simulink model "chap7_4sim"  (Simulink 3.00)
settings: Solver=ode45  StartTime=0.0  StopTime=50  FixedStep=0.00001  RelTol=1e-3
settings Model: LastModifiedBy=liu

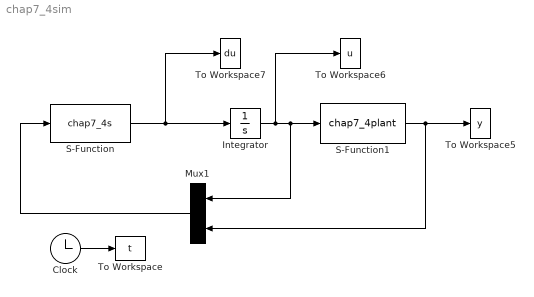
== system chap7_4sim ==
  Clock : Clock
  Integrator : Integrator  ExternalReset=none  InitialConditionSource=internal  InitialCondition=0  LimitOutput=off  UpperSaturationLimit=inf  LowerSaturationLimit=-inf  ShowSaturationPort=off  ShowStatePort=off  AbsoluteTolerance=auto
  Mux1 : Mux  Orientation=left  Inputs=2
  S-Function : S-Function  FunctionName=chap7_4s  PortCounts=[]  SFunctionModules=''
  S-Function1 : S-Function  FunctionName=chap7_4plant  PortCounts=[]  SFunctionModules=''
  To Workspace : ToWorkspace  VariableName=t  SampleTime=-1  SaveFormat=Matrix
  To Workspace5 : ToWorkspace  VariableName=y  SampleTime=-1  SaveFormat=Matrix
  To Workspace6 : ToWorkspace  VariableName=u  SampleTime=-1  SaveFormat=Matrix
  To Workspace7 : ToWorkspace  VariableName=du  SampleTime=-1  SaveFormat=Matrix
  wires:
  S-Function1/1 -> To Workspace5/1, Mux1/2
  Integrator/1 -> S-Function1/1, Mux1/1, To Workspace6/1
  Mux1/1 -> S-Function/1
  S-Function/1 -> Integrator/1, To Workspace7/1
  Clock/1 -> To Workspace/1
